simulink model "CTRL_TRGT_DEC_test"  (R2023b)
settings: Solver=VariableStepAuto  StartTime=0.0  StopTime=10.0  RelTol=1e-3
libraries: CTRL_TRGT_DEC x1
settings Model: Creator=blatak  LastModifiedBy=blatak

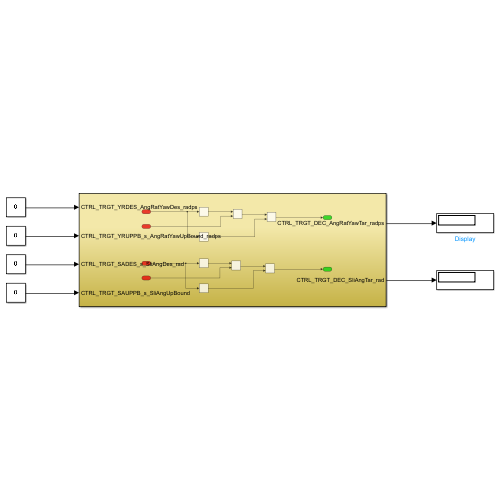
[thumbnail: Simulink's stored preview of the top-level diagram]
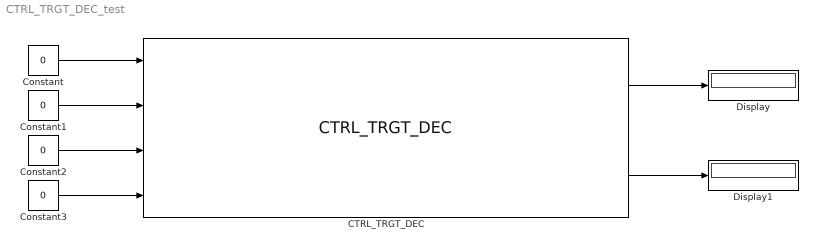
== system CTRL_TRGT_DEC_test ==
  CTRL_TRGT_DEC : CTRL_TRGT_DEC/CTRL_TRGT_DEC  SystemSampleTime=-1  VariantActivationTime=update diagram  AllowFlexibleInterface=on  Latency=0  AutoFrameSizeCalculation=off
  Constant{,1..3} (4 alike) : Constant  Value=0  OutDataTypeStr=single
  Display : Display
  Display1 : Display
  wires:
  Constant/1 -> CTRL_TRGT_DEC/1
  Constant1/1 -> CTRL_TRGT_DEC/2
  Constant2/1 -> CTRL_TRGT_DEC/3
  Constant3/1 -> CTRL_TRGT_DEC/4
  CTRL_TRGT_DEC/1 -> Display/1
  CTRL_TRGT_DEC/2 -> Display1/1
